simulink model "Test2"  (R2022b)
settings: Solver=ode1  StartTime=0.0  StopTime=inf  FixedStep=0.002  RelTol=1e-3  EnableMultiTasking=on
PostLoadFcn:
  | qc_set_target_type(getConfigSet(bdroot, 'QUARC Default Target Configuration'));
undefined symbols (not defined in the file or in its folder): HIL, qc_get_step_size
libraries: quarc_library x8, simulink_extras x4, simulink x2
settings Model: SimulationMode=external  ExtModeTrigDuration=10000  Creator=CFulford  LastModifiedBy=Utente
settings SolverCC: AlgebraicLoopSolver=TrustRegion  PositivePriorityOrder=on
settings DataIOCC: LimitDataPoints=on  SaveFormat=Array  SignalLoggingSaveFormat=ModelDataLogs  ReturnWorkspaceOutputs=off
settings OptimizationCC: ExpressionDepthLimit=2147483647  InitFltsAndDblsToZero=on
settings DebuggingCC: SaveWithParameterizedLinksMsg=none  UnderspecifiedInitializationDetection=Classic  MergeDetectMultiDrivingBlocksExec=none  SolverPrmCheckMsg=warning  MultiTaskDSMMsg=warning  MultiTaskCondExecSysMsg=none  FcnCallInpInsideContextMsg=warning  UnconnectedInputMsg=warning  UnconnectedOutputMsg=warning  UnconnectedLineMsg=warning  StateNameClashWarn=warning  SFUnexpectedBacktrackingDiag=warning  SFNoUnconditionalDefaultTransitionDiag=warning  SFExecutionAtInitializationDiag=none  SFMachineParentedDataDiag=warning  ArithmeticOperatorsInVariantConditions=warning
settings ModelReferenceCC: EnableRefExpFcnMdlSchedulingChecks=on  PropagateSignalLabelsOutOfModel=off
settings SFSimCC: SimUseLocalCustomCode=off  CustomCodeUndefinedFunction=UseInterfaceOnly
settings RTWCC: Description=QUARC Win64 Target Using Toolchain  SystemTargetFile=quarc_win64.tlc  TemplateMakefile=quarc_default_tmf  RTWUseLocalCustomCode=off  Toolchain=QUARC win64 | nmake (64-bit Windows)  BuildConfiguration=Faster Runs
settings CodeAppCC: StateflowObjectComments=on
settings STFCustomTargetCC: ConcurrentExecutionCompliant=on  GRTInterface=on  UseToolchainInfoCompliant=on  SystemTargetFile=quarc_win64.tlc
settings GRTTargetCC: TargetLangStandard=C89/C90 (ANSI)  ParMdlRefBuildCompliant=off  CompOptLevelCompliant=off  CombineOutputUpdateFcns=off  MatFileLogging=off  CPPClassGenCompliant=off  GRTInterface=on  ExtMode=on  ExtModeMexFile=quarc_comm
settings ConfigComp: CovMetricSettings=dw  CovSaveCumulativeToWorkspaceVar=on  CovSaveSingleToWorkspaceVar=on  CovExternalEMLEnable=off  CovSFcnEnable=off

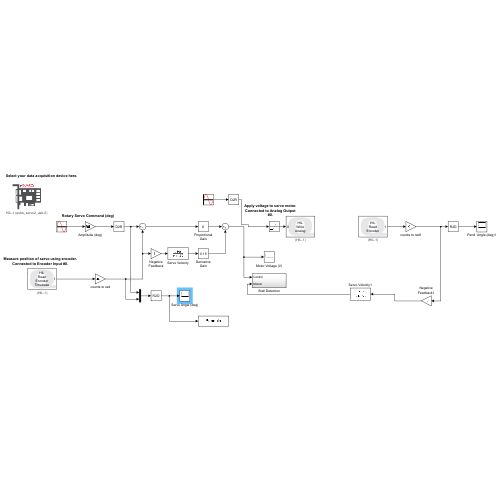
[thumbnail: Simulink's stored preview of the top-level diagram]
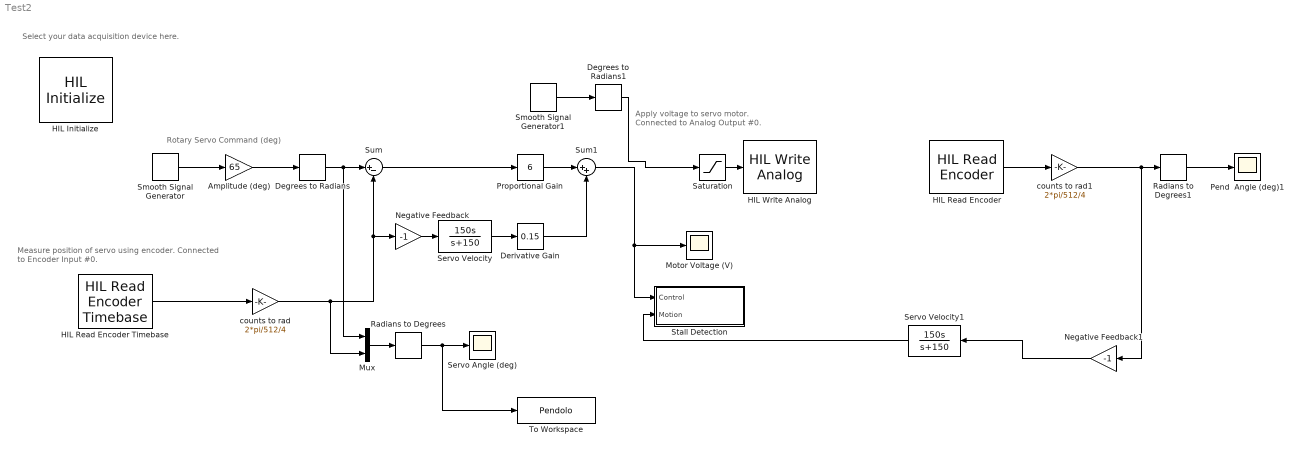
== system Test2 ==
  note: Rotary Servo Command (deg)
  note: Apply voltage to servo motor.
      | Connected to Analog Output #0.
  note: Measure position of servo using encoder.
      | Connected to Encoder Input #0.
  note: Select your data acquisition device here.
  Amplitude (deg) : Gain  Gain=65
  Degrees to Radians : simulink_extras/Transformations/Degrees to Radians
  Degrees to Radians1 : simulink_extras/Transformations/Degrees to Radians
  Derivative Gain : simulink/Math Operations/Slider Gain  gain=0.15  low=0  high=0.5
  HIL Initialize : quarc_library/Data Acquisition/Generic/Configuration/HIL Initialize  Priority=-99  object_name=HIL-1  board_type=qube_servo2_usb  board_number=0  board_options=""  exclusive=off  active=off  hardware_clocks=[0]  clock_modes=[]  initial_clock_frequencies=[]  set_clock_params_at_start=off  set_clock_params_at_switch_in=off  set_clock_frequencies_at_start=off  set_clock_frequencies_at_switch_in=off  analog_input_channels=[0]  analog_input_configurations=[]  analog_input_maximums=3  analog_input_minimums=-3  set_analog_input_params_at_start=off  set_analog_input_params_at_switch_in=off  analog_output_channels=[0]  analog_output_maximums=15  analog_output_minimums=-15  initial_analog_outputs=[0]  final_analog_outputs=[0]  watchdog_analog_outputs=0  set_analog_output_params_at_start=off  set_analog_output_params_at_switch_in=off  set_analog_outputs_at_start=on  set_analog_outputs_at_switch_in=off  set_analog_outputs_at_terminate=on  set_analog_outputs_at_switch_out=off  set_analog_outputs_on_watchdog=on  digital_input_channels=[]  digital_output_channels=[0]  digital_output_configuration=[]  initial_digital_outputs=[1]  final_digital_outputs=[0]  watchdog_digital_outputs=[0]  set_digital_output_params_at_start=off  set_digital_output_params_at_switch_in=off  set_digital_outputs_at_start=on  set_digital_outputs_at_switch_in=off  set_digital_outputs_at_terminate=on  set_digital_outputs_at_switch_out=off  set_digital_outputs_on_watchdog=on  encoder_channels=[0:1]  quadrature=[4]  encoder_filter_frequency=[]  initial_encoder_counts=[0]  set_encoder_params_at_start=off  set_encoder_params_at_switch_in=off  set_encoder_counts_at_start=on  set_encoder_counts_at_switch_in=off  pwm_channels=[]  pwm_modes=[]  pwm_frequency=[]  pwm_configuration=[]  pwm_alignment=[]  pwm_polarity=[]  pwm_leading_deadband=[]  pwm_trailing_deadband=[]  initial_pwm_outputs=[]  final_pwm_outputs=[]  watchdog_pwm_outputs=[]  set_pwm_params_at_start=off  set_pwm_params_at_switch_in=off  set_pwm_outputs_at_start=off  set_pwm_outputs_at_switch_in=off  set_pwm_outputs_at_terminate=off  set_pwm_outputs_at_switch_out=off  set_pwm_outputs_on_watchdog=off  other_output_channels=[11000:11002]  initial_other_outputs=[0 1 0]  final_other_outputs=[1 0 0]  watchdog_other_outputs=[0 0 1]  set_other_outputs_at_start=on  set_other_outputs_at_switch_in=off  set_other_outputs_at_terminate=on  set_other_outputs_at_switch_out=off  set_other_outputs_on_watchdog=on
  HIL Read Encoder : quarc_library/Data Acquisition/Generic/Immediate I//O/HIL Read Encoder  object_name=HIL-1  channels=[1]  sample_time=qc_get_step_size  active=on  vector_output=off  data_type_mode=Inherit via back propagation  data_type=double
  HIL Read Encoder Timebase : quarc_library/Data Acquisition/Generic/Timebases/HIL Read Encoder Timebase  object_name=HIL-1  clock=0  channels=1  active=on  vector_output=off  data_type_mode=Inherit via back propagation  data_type=double  overflow_mode=Error on overflow  samples_in_buffer=max(ceil(1/qc_get_step_size), 1)
  HIL Write Analog : quarc_library/Data Acquisition/Generic/Immediate I//O/HIL Write Analog  object_name=HIL-1  channels=0  sample_time=-1  active=off  vector_input=off
  Motor Voltage (V) : Scope
  Mux : Mux  Inputs=2
  Negative Feedback : Gain  Gain=-1
  Negative Feedback1 : Gain  Gain=-1
  Pend  Angle (deg)1 : Scope
  Proportional Gain : simulink/Math Operations/Slider Gain  gain=6  low=0  high=10
  Radians to Degrees : simulink_extras/Transformations/Radians to Degrees
  Radians to Degrees1 : simulink_extras/Transformations/Radians to Degrees
  Saturation : Saturate  UpperLimit=5  LowerLimit=-5
  Servo Angle (deg) : Scope
  Servo Velocity : TransferFcn  Numerator=[150 0]  Denominator=[1 150]
  Servo Velocity1 : TransferFcn  Numerator=[150 0]  Denominator=[1 150]
  Smooth Signal Generator : quarc_library/Sources/Signals/Smooth Signal Generator  signal_type=Sine  source=Internal (dialog parameters)  amplitude=0  frequency=2.5  initial_phase=-pi/4  sample_time=qc_get_step_size  output_cos=off
      settings: SourceProductName=QUARC Targets
  Smooth Signal Generator1 : quarc_library/Sources/Signals/Smooth Signal Generator  signal_type=Sine  source=Internal (dialog parameters)  amplitude=0  frequency=2.5  initial_phase=-pi/4  sample_time=qc_get_step_size  output_cos=off
      settings: SourceProductName=QUARC Targets
  Stall Detection : Subsystem
  Sum : Sum  Inputs=|+-
  Sum1 : Sum  Inputs=|++
  To Workspace : ToWorkspace  VariableName=Pendolo  SampleTime=-1
  counts to rad : Gain  Gain=2*pi/512/4
  counts to rad1 : Gain  Gain=2*pi/512/4
  wires:
  Sum/1 -> Proportional Gain/1
  counts to rad/1 -> Sum/2, Negative Feedback/1, Mux/2
  Proportional Gain/1 -> Sum1/1
  Servo Velocity/1 -> Derivative Gain/1
  Derivative Gain/1 -> Sum1/2
  Smooth Signal Generator/1 -> Amplitude (deg)/1
  Amplitude (deg)/1 -> Degrees to Radians/1
  Degrees to Radians/1 -> Sum/1, Mux/1
  Negative Feedback/1 -> Servo Velocity/1
  Mux/1 -> Radians to Degrees/1
  Radians to Degrees/1 -> To Workspace/1, Servo Angle (deg)/1
  HIL Read Encoder Timebase/1 -> counts to rad/1
  HIL Read Encoder/1 -> counts to rad1/1
  Radians to Degrees1/1 -> Pend  Angle (deg)1/1
  counts to rad1/1 -> Negative Feedback1/1, Radians to Degrees1/1
  Sum1/1 -> Stall Detection/1(Control), Motor Voltage (V)/1
  Saturation/1 -> HIL Write Analog/1
  Negative Feedback1/1 -> Servo Velocity1/1
  Servo Velocity1/1 -> Stall Detection/2(Motion)
  Smooth Signal Generator1/1 -> Degrees to Radians1/1
  Degrees to Radians1/1 -> Saturation/1

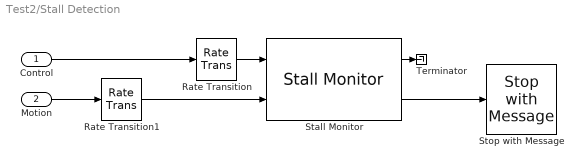
== system Test2/Stall Detection ==
  Control : Inport
  Motion : Inport  Port=2
  Rate Transition : RateTransition
  Rate Transition1 : RateTransition
  Stall Monitor : quarc_library/Discrete/Stall Monitor  control_threshold=5  motion_threshold=0.3  duration_s=20
      settings: SourceProductName=QUARC Targets
  Stop with Message : quarc_library/Sinks/Error Handling/Stop with Message  message_type=Fixed error message  message_icon=Error  message=Stall Detected! Please ensure that the DC motor is free to move and is functioning properly
  Terminator : Terminator
  wires:
  Control/1 -> Rate Transition/1
  Motion/1 -> Rate Transition1/1
  Stall Monitor/2 -> Stop with Message/1
  Stall Monitor/1 -> Terminator/1
  Rate Transition/1 -> Stall Monitor/1
  Rate Transition1/1 -> Stall Monitor/2
